simulink model "MotDynoReferenceApplication"  (R2023a)
settings: Solver=VariableStepAuto  StartTime=0.0  StopTime=36  RelTol=1e-3
libraries: simulink x2, autolibinverter x2, autolibmotorctrlr x2, autolibpowerinfoutils x1, autolibpmsminterior x1, autolibfluxpmsm x1, autolibmappedmotor x1
(part 3 of 7)

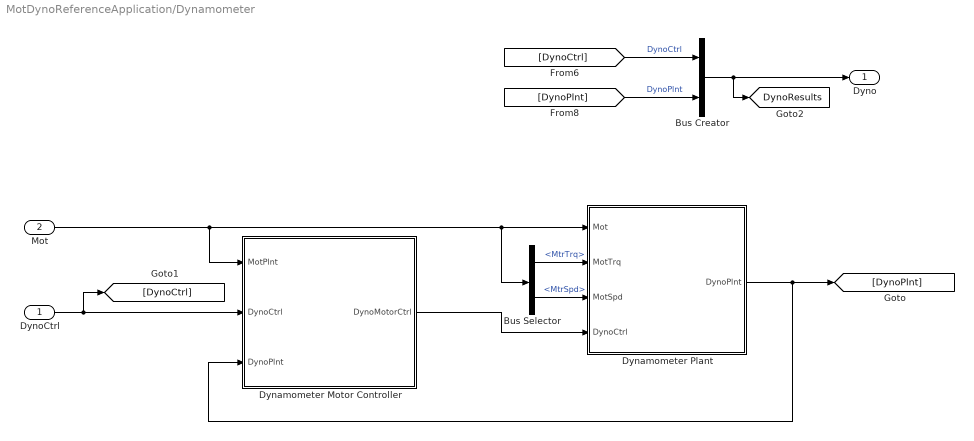
== system MotDynoReferenceApplication/Dynamometer ==
  DynoCtrl : Inport
  Mot : Inport  Port=2
  Bus Creator : BusCreator  Inputs=2
  Bus Selector : BusSelector  OutputSignals=MotPlnt.MtrTrq,MotPlnt.MtrSpd
  Dynamometer Motor Controller : Subsystem
  Dynamometer Plant : Subsystem
  Dyno : Outport  VectorParamsAs1DForOutWhenUnconnected=off
  tag scope: DynoResults=global
  wires:
  Bus Creator/1 -> Dyno/1, [DynoResults]
  Mot/1 -> Bus Selector/1, Dynamometer Plant/1(Mot), Dynamometer Motor Controller/1(MotPlnt)
  Dynamometer Plant/1(DynoPlnt) -> [DynoPlnt], Dynamometer Motor Controller/3(DynoPlnt)
  Dynamometer Motor Controller/1(DynoMotorCtrl) -> Dynamometer Plant/4(DynoCtrl)
  [DynoPlnt] -> Bus Creator/2  "DynoPlnt"
  [DynoCtrl] -> Bus Creator/1  "DynoCtrl"
  DynoCtrl/1 -> [DynoCtrl], Dynamometer Motor Controller/2(DynoCtrl)
  Bus Selector/1 -> Dynamometer Plant/2(MotTrq)  "<MtrTrq>"
  Bus Selector/2 -> Dynamometer Plant/3("MotSpd ")  "<MtrSpd>"

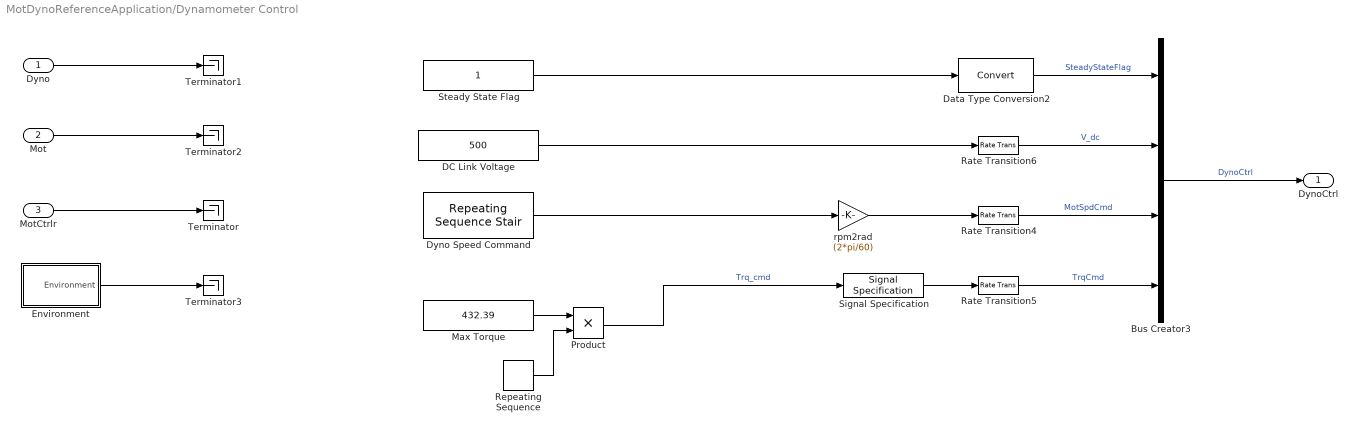
== system MotDynoReferenceApplication/Dynamometer Control ==
  Dyno : Inport
  Mot : Inport  Port=2
  MotCtrlr : Inport  Port=3
  Bus Creator3 : BusCreator  Inputs=4
  DC Link Voltage : Constant  Value=500
  Data Type Conversion2 : DataTypeConversion  SaturateOnIntegerOverflow=off  RndMeth=Floor
  Dyno Speed Command : simulink/Sources/Repeating Sequence Stair  OutValues=[500;1000;1500;2000;2500;3000;3500;4000;4500;5000;5500;6000]  tsamp=3  OutMin=[]  OutMax=[]  OutDataTypeStr=double  OutputDataTypeScalingMode=double  OutDataType=fixdt(0,8)  ConRadixGroup=Best Precision: Vector-wise  OutScaling=2^-12
  Environment : Subsystem
  Max Torque : Constant  Value=432.39
  Product : Product
  Rate Transition4 : RateTransition  Deterministic=off
  Rate Transition5 : RateTransition
  Rate Transition6 : RateTransition  Deterministic=off
  Repeating Sequence : simulink/Sources/Repeating Sequence  rep_seq_t=[0 2 3]  rep_seq_y=[0 1 0]
  Signal Specification : SignalSpecification  Unit=N*m
  Steady State Flag : Constant
  Terminator{,1..3} (4 alike) : Terminator
  rpm2rad : Gain  Gain=(2*pi/60)
  DynoCtrl : Outport  VectorParamsAs1DForOutWhenUnconnected=off
  wires:
  Bus Creator3/1 -> DynoCtrl/1  "DynoCtrl"
  Data Type Conversion2/1 -> Bus Creator3/1  "SteadyStateFlag"
  Rate Transition6/1 -> Bus Creator3/2  "V_dc"
  Rate Transition5/1 -> Bus Creator3/4  "TrqCmd"
  Rate Transition4/1 -> Bus Creator3/3  "MotSpdCmd"
  Dyno/1 -> Terminator1/1
  Mot/1 -> Terminator2/1
  Signal Specification/1 -> Rate Transition5/1
  DC Link Voltage/1 -> Rate Transition6/1
  MotCtrlr/1 -> Terminator/1
  Steady State Flag/1 -> Data Type Conversion2/1
  rpm2rad/1 -> Rate Transition4/1
  Environment/1(Environment) -> Terminator3/1
  Repeating Sequence/1 -> Product/2
  Product/1 -> Signal Specification/1  "Trq_cmd"
  Max Torque/1 -> Product/1
  Dyno Speed Command/1 -> rpm2rad/1

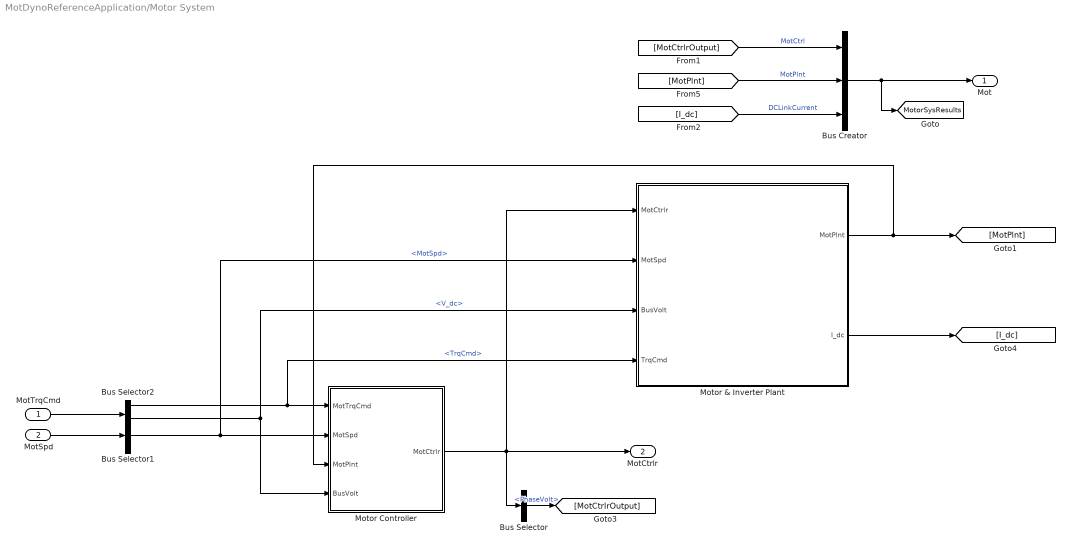
== system MotDynoReferenceApplication/Motor System ==
  MotTrqCmd : Inport
  MotSpd : Inport  Port=2
  Bus Creator : BusCreator  Inputs=3
  Bus Selector : BusSelector  OutputSignals=PhaseVolt
  Bus Selector1 : BusSelector  OutputSignals=DynoPlnt.MotSpd
  Bus Selector2 : BusSelector  OutputSignals=TrqCmd,V_dc
  Motor & Inverter Plant : Subsystem  Variant=on  VariantControlMode=label  LabelModeActiveChoice=Flux-Based PMSM Model
  Motor Controller : Subsystem  Variant=on  VariantControlMode=label  LabelModeActiveChoice=Flux-Based PMSM Model
  Mot : Outport  VectorParamsAs1DForOutWhenUnconnected=off
  MotCtrlr : Outport  Port=2  VectorParamsAs1DForOutWhenUnconnected=off
  tag scope: MotorSysResults=global
  wires:
  Bus Selector2/2 -> Motor Controller/4(BusVolt), Motor & Inverter Plant/3(BusVolt)  "<V_dc>"
  Bus Selector1/1 -> Motor Controller/2(MotSpd), Motor & Inverter Plant/2(MotSpd)  "<MotSpd>"
  Motor & Inverter Plant/1(MotPlnt) -> Motor Controller/3(MotPlnt), [MotPlnt]
  Bus Creator/1 -> Mot/1, [MotorSysResults]
  [MotPlnt] -> Bus Creator/2  "MotPlnt"
  [MotCtrlrOutput] -> Bus Creator/1  "MotCtrl"
  Motor Controller/1(MotCtrlr) -> Bus Selector/1, Motor & Inverter Plant/1(MotCtrlr), MotCtrlr/1
  [I_dc] -> Bus Creator/3  "DCLinkCurrent"
  Bus Selector2/1 -> Motor & Inverter Plant/4(TrqCmd), Motor Controller/1(MotTrqCmd)  "<TrqCmd>"
  Motor & Inverter Plant/2(I_dc) -> [I_dc]
  MotTrqCmd/1 -> Bus Selector2/1
  MotSpd/1 -> Bus Selector1/1
  Bus Selector/1 -> [MotCtrlrOutput]  "<PhaseVolt>"

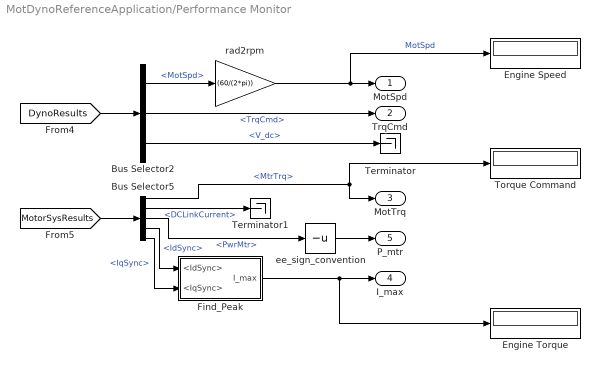
== system MotDynoReferenceApplication/Performance Monitor ==
  Bus Selector2 : BusSelector  OutputSignals=DynoPlnt.MotSpd,DynoCtrl.TrqCmd,DynoCtrl.V_dc
  Bus Selector5 : BusSelector  OutputSignals=MotPlnt.MtrTrq,DCLinkCurrent,MotPlnt.PwrInfo.PwrTrnsfrd.PwrMtr,MotPlnt.IdSync,MotPlnt.IqSync
  Engine Speed : Display
      settings: Decimation=100
  Engine Torque : Display
      settings: Decimation=100
  Find_Peak : Subsystem
  Terminator : Terminator
  Terminator1 : Terminator
  Torque Command : Display
      settings: Decimation=100
  ee_sign_convention : UnaryMinus
  rad2rpm : Gain  Gain=(60/(2*pi))
  MotSpd : Outport  VectorParamsAs1DForOutWhenUnconnected=off
  TrqCmd : Outport  Port=2  VectorParamsAs1DForOutWhenUnconnected=off
  MotTrq : Outport  Port=3  VectorParamsAs1DForOutWhenUnconnected=off
  I_max : Outport  Port=4  VectorParamsAs1DForOutWhenUnconnected=off
  P_mtr : Outport  Port=5  VectorParamsAs1DForOutWhenUnconnected=off
  wires:
  Bus Selector5/1 -> MotTrq/1, Torque Command/1  "<MtrTrq>"
  [MotorSysResults] -> Bus Selector5/1
  Bus Selector2/2 -> TrqCmd/1  "<TrqCmd>"
  rad2rpm/1 -> Engine Speed/1, MotSpd/1  "MotSpd"
  [DynoResults] -> Bus Selector2/1
  Bus Selector2/3 -> Terminator/1  "<V_dc>"
  Bus Selector2/1 -> rad2rpm/1  "<MotSpd>"
  Bus Selector5/3 -> ee_sign_convention/1  "<PwrMtr>"
  Bus Selector5/2 -> Terminator1/1  "<DCLinkCurrent>"
  Find_Peak/1(I_max) -> Engine Torque/1, I_max/1
  Bus Selector5/4 -> Find_Peak/1(<IdSync>)  "<IdSync>"
  Bus Selector5/5 -> Find_Peak/2(<IqSync>)  "<IqSync>"
  ee_sign_convention/1 -> P_mtr/1

== system MotDynoReferenceApplication/Resize Dynamic PMSMs ==
  note: Note:
      | This is a floating block.
  Constant : Constant
  Terminator : Terminator
  wires:
  Constant/1 -> Terminator/1

== system MotDynoReferenceApplication/Resize Flux-based PMSMs ==
  note: Note:
      | This is a floating block.
  Constant : Constant
  Terminator : Terminator
  wires:
  Constant/1 -> Terminator/1

== system MotDynoReferenceApplication/Resize Mapped Motors ==
  note: Note:
      | This is a floating block.
  Constant : Constant
  Terminator : Terminator
  wires:
  Constant/1 -> Terminator/1

== system MotDynoReferenceApplication/Run Performance Tests ==
  note: Note:
      | This is a floating block.
  Constant : Constant
  Terminator : Terminator
  wires:
  Constant/1 -> Terminator/1

== system MotDynoReferenceApplication/Subsystem4 ==

== system MotDynoReferenceApplication/Dynamometer/Dynamometer Motor Controller ==
  MotPlnt : Inport
  DynoCtrl : Inport  Port=2
  DynoPlnt : Inport  Port=3
  Bus Creator : BusCreator  Inputs=2
  Bus Selector : BusSelector  OutputSignals=MotSpdCmd,SteadyStateFlag
  Terminator : Terminator
  Terminator1 : Terminator
  DynoMotorCtrl : Outport  VectorParamsAs1DForOutWhenUnconnected=off
  wires:
  DynoCtrl/1 -> Bus Selector/1
  MotPlnt/1 -> Terminator/1
  DynoPlnt/1 -> Terminator1/1
  Bus Selector/1 -> Bus Creator/1  "<MotSpdCmd>"
  Bus Creator/1 -> DynoMotorCtrl/1
  Bus Selector/2 -> Bus Creator/2  "<SteadyStateFlag>"

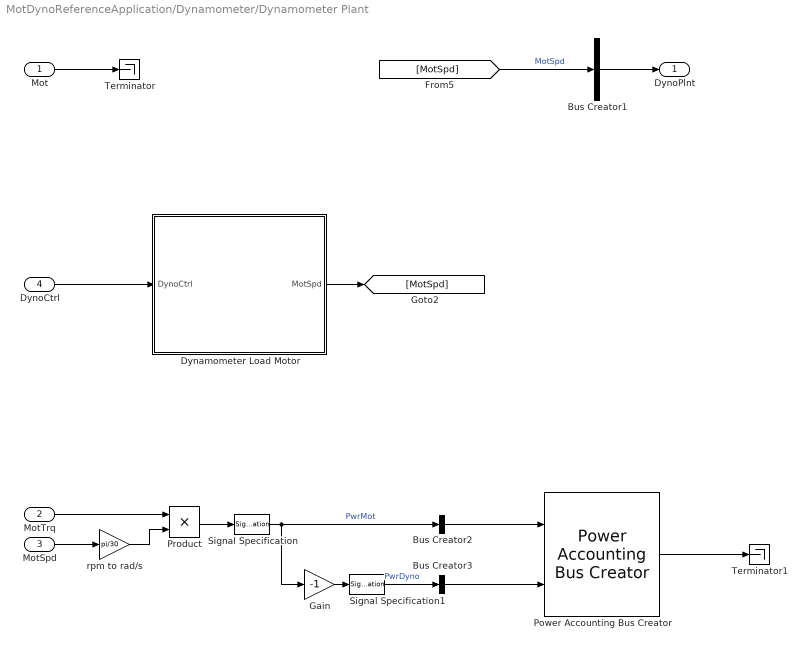
== system MotDynoReferenceApplication/Dynamometer/Dynamometer Plant ==
  Mot : Inport
  MotTrq : Inport  Port=2
  "MotSpd " : Inport  Port=3
  DynoCtrl : Inport  Port=4
  Bus Creator1 : BusCreator  Inputs=1
  Bus Creator2 : BusCreator  Inputs=1
  Bus Creator3 : BusCreator  Inputs=1
  Dynamometer Load Motor : Subsystem
  Gain : Gain  Gain=-1
  Power Accounting Bus Creator : autolibpowerinfoutils/Power Accounting Bus Creator  AssctBlkSelPopup=Parent  RefBlkName='libraryname/blkname'  PwrTrnsfrdCheckBox=on  PwrNotTrnsfrdCheckBox=on  PwrStoredCheckBox=off  aMode=aMode
  Product : Product
  Signal Specification : SignalSpecification  Unit=W
  Signal Specification1 : SignalSpecification  Unit=W
  Terminator : Terminator
  Terminator1 : Terminator
  rpm to rad/s : Gain  Gain=pi/30
  DynoPlnt : Outport  VectorParamsAs1DForOutWhenUnconnected=off
  wires:
  Dynamometer Load Motor/1(MotSpd) -> [MotSpd]
  Bus Creator1/1 -> DynoPlnt/1
  [MotSpd] -> Bus Creator1/1  "MotSpd"
  DynoCtrl/1 -> Dynamometer Load Motor/1(DynoCtrl)
  Mot/1 -> Terminator/1
  Bus Creator2/1 -> Power Accounting Bus Creator/1
  Signal Specification/1 -> Gain/1, Bus Creator2/1  "PwrMot"
  Bus Creator3/1 -> Power Accounting Bus Creator/2
  Power Accounting Bus Creator/1 -> Terminator1/1
  Gain/1 -> Signal Specification1/1
  Product/1 -> Signal Specification/1
  Signal Specification1/1 -> Bus Creator3/1  "PwrDyno"
  MotTrq/1 -> Product/1
  "MotSpd "/1 -> rpm to rad/s/1
  rpm to rad/s/1 -> Product/2

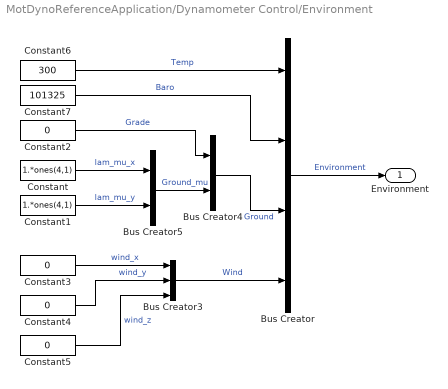
== system MotDynoReferenceApplication/Dynamometer Control/Environment ==
  Bus Creator : BusCreator  Inputs=4
  Bus Creator3 : BusCreator  Inputs=3
  Bus Creator4 : BusCreator  Inputs=2
  Bus Creator5 : BusCreator  Inputs=2
  Constant : Constant  Value=1.*ones(4,1)
  Constant1 : Constant  Value=1.*ones(4,1)
  Constant{2..5} (4 alike) : Constant  Value=0
  Constant6 : Constant  Value=300
  Constant7 : Constant  Value=101325
  Environment : Outport  VectorParamsAs1DForOutWhenUnconnected=off
  wires:
  Constant/1 -> Bus Creator5/1  "lam_mu_x"
  Constant1/1 -> Bus Creator5/2  "lam_mu_y"
  Bus Creator5/1 -> Bus Creator4/2  "Ground_mu"
  Bus Creator4/1 -> Bus Creator/3  "Ground"
  Bus Creator3/1 -> Bus Creator/4  "Wind"
  Constant3/1 -> Bus Creator3/1  "wind_x"
  Constant4/1 -> Bus Creator3/2  "wind_y"
  Constant5/1 -> Bus Creator3/3  "wind_z"
  Constant6/1 -> Bus Creator/1  "Temp"
  Constant2/1 -> Bus Creator4/1  "Grade"
  Bus Creator/1 -> Environment/1  "Environment"
  Constant7/1 -> Bus Creator/2  "Baro"

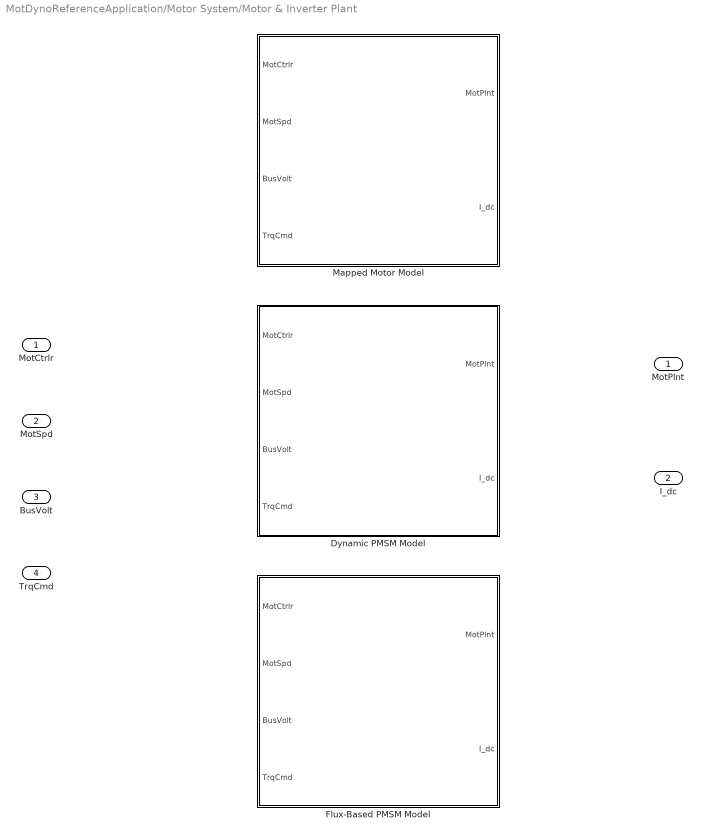
== system MotDynoReferenceApplication/Motor System/Motor & Inverter Plant ==
  MotCtrlr : Inport
  MotSpd : Inport  Port=2
  BusVolt : Inport  Port=3
  TrqCmd : Inport  Port=4
  Dynamic PMSM Model : Subsystem  VariantControl=Dynamic Motor Model
  Flux-Based PMSM Model : Subsystem  VariantControl=Flux-Based PMSM Model
  Mapped Motor Model : Subsystem  VariantControl=Mapped Motor Model
  MotPlnt : Outport  VectorParamsAs1DForOutWhenUnconnected=off
  I_dc : Outport  Port=2  VectorParamsAs1DForOutWhenUnconnected=off

== system MotDynoReferenceApplication/Motor System/Motor Controller ==
  MotTrqCmd : Inport
  MotSpd : Inport  Port=2
  MotPlnt : Inport  Port=3
  BusVolt : Inport  Port=4
  Flux-Based PM Controller : Subsystem  VariantControl=Flux-Based PMSM Model
  Interior PM Controller SS Trq : Subsystem  VariantControl=Dynamic Motor Model
  Mapped Motor Controller : Subsystem  VariantControl=Mapped Motor Model
  MotCtrlr : Outport  VectorParamsAs1DForOutWhenUnconnected=off

== system MotDynoReferenceApplication/Performance Monitor/Find_Peak ==
  <IdSync> : Inport
  <IqSync> : Inport  Port=2
  Sqrt : Sqrt
  Square : Math  Operator=square
  Square1 : Math  Operator=square
  Sum : Sum  Inputs=|++
  I_max : Outport
  wires:
  Sqrt/1 -> I_max/1  "I_max"
  Sum/1 -> Sqrt/1
  <IdSync>/1 -> Square/1
  Square/1 -> Sum/1
  Square1/1 -> Sum/2
  <IqSync>/1 -> Square1/1

== system MotDynoReferenceApplication/Dynamometer/Dynamometer Plant/Dynamometer Load Motor ==
  DynoCtrl : Inport
  Bus Selector : BusSelector  OutputSignals=MotSpdCmd
  Dyno Dynamics : TransferFcn  Denominator=[0.1 1]
  MotSpd : Outport  VectorParamsAs1DForOutWhenUnconnected=off
  wires:
  Dyno Dynamics/1 -> MotSpd/1
  DynoCtrl/1 -> Bus Selector/1
  Bus Selector/1 -> Dyno Dynamics/1  "<MotSpdCmd>"

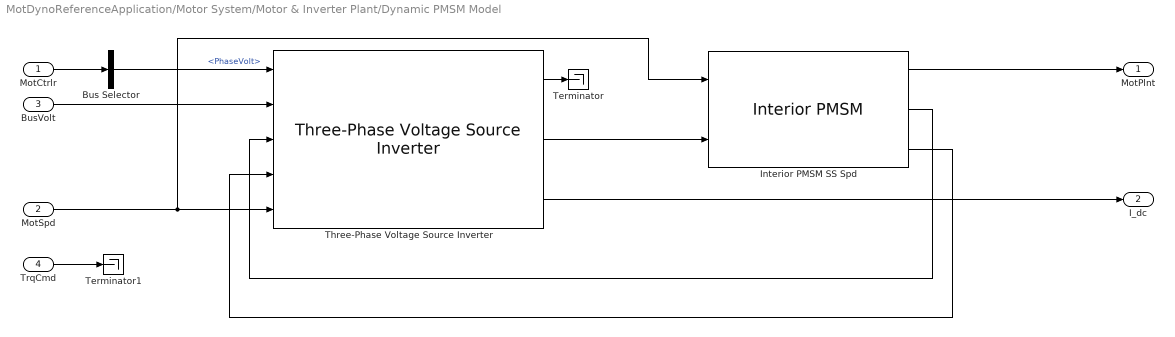
== system MotDynoReferenceApplication/Motor System/Motor & Inverter Plant/Dynamic PMSM Model ==
  MotCtrlr : Inport
  MotSpd : Inport  Port=2
  BusVolt : Inport  Port=3
  TrqCmd : Inport  Port=4
  Bus Selector : BusSelector  OutputSignals=PhaseVolt
  Interior PMSM SS Spd : autolibpmsminterior/Interior PMSM  VariantControl=Dynamic Motor Model  port_config=Speed  sim_type=Continuous  Ts=0.001  P=4  Rs=0.0096  Ldq=[0.00024276 0.00036413]  KConstText=Permanent flux linkage constant (lambda_pm):  lambda_pm=0.1331  Ke=159.9771  mechanical=mechanical  idq0=[0 0]  theta_init=0  omega_init=omega_init  KConst=0.1331  lambda_pm_calc=0.1331  Kt=1.323  RefBlkName='autolibpmsminterior/Interior PMSM'  aMode=1
      settings: LibrarySourceBlock=autolibemachines/Interior PMSM
  Terminator : Terminator
  Terminator1 : Terminator
  Three-Phase Voltage Source Inverter : autolibinverter/Three-Phase Voltage Source Inverter  InvrtrTmpInpEnbl=off  enable_hdl=off  model_type=Commanded phase voltage  fs=5000  w_eff_bp=[-1000 -500 0 500 1000]  n1=128  T_eff_bp=[-100 -50 0 50 100]*450  Temp_eff_bp=[213.15 293.15 373.15]  n2=128  ploss_table=0.98*ones(5,5)  ploss_table_3d=cat(3,0.95*[1 0.999 0.989 0.997 0.996;0.995 0.994 0.993 0.992 0.991;0.990 0.989 0.988 0.987 0.986;0.985 0.984 0.983 0.982 0.981;0.980 0.979 0.978 0.977 0.976],[1 0.999 0.989 0.997 0.996;0.995 0.994 0.993 0.992 0.991;0.990 0.989 0.988 0.987 0.986;0.985 0.984 0.983 0.982 0.981;0.980 0.979 0.978 0.977 0.976],0.92*[1 0.999 0.989 0.997 0.996;0.995 0.994 0.993 0.992 0.991;0.990 0.989 0.988 0.987 0.986;0.985 0.984 0.983 0.982 0.981;0.980 0.979 0.978 0.977 0.976])  preExtrapFlag=off  u1max=1000  u1min=-1000  u2max=200  u2min=-200  intPrec=23  RefBlkName='autolibmappedmotor/Mapped Motor'  CalLossMapData={}  CalLossWithTempMapData={}
  MotPlnt : Outport  VectorParamsAs1DForOutWhenUnconnected=off
  I_dc : Outport  Port=2  VectorParamsAs1DForOutWhenUnconnected=off
  wires:
  Three-Phase Voltage Source Inverter/3 -> I_dc/1
  Three-Phase Voltage Source Inverter/2 -> Interior PMSM SS Spd/2
  Three-Phase Voltage Source Inverter/1 -> Terminator/1
  Interior PMSM SS Spd/2 -> Three-Phase Voltage Source Inverter/3
  Interior PMSM SS Spd/3 -> Three-Phase Voltage Source Inverter/4
  MotCtrlr/1 -> Bus Selector/1
  MotSpd/1 -> Interior PMSM SS Spd/1, Three-Phase Voltage Source Inverter/5
  Interior PMSM SS Spd/1 -> MotPlnt/1
  BusVolt/1 -> Three-Phase Voltage Source Inverter/2
  Bus Selector/1 -> Three-Phase Voltage Source Inverter/1  "<PhaseVolt>"
  TrqCmd/1 -> Terminator1/1
